simulink model "heli_model"  (R2025a)
settings: Solver=ode3  StartTime=0.0  StopTime=300  FixedStep=0.001
values from neighbouring files (symbols this model uses):
  alt = -1000    [Trim_Lin_Lqr.m]
  Vrefs = [15 20 25]    [Trim_Lin_Lqr.m]
  wp = [0 0; 1000 1000; 2000 0; 1000 -1000; 0 -100]    [Trim_Lin_Lqr.m]
undefined symbols (not defined in the file or in its folder): AngVel, AngVeltr, Coeffs, Lfin, LQR, MTOW, R, rad, Rtr, s
libraries: slpidlib x2, simulink x2, aerolibatmos2 x2, matrix_library x2, aerolibconvert2 x2, aerolibfltsims x2, aerolibsim3d x2, aerolibobsolete x1, sim3dlib x1
settings Model: PacingRate=1000  Creator=stand-alone1  LastModifiedBy=celal

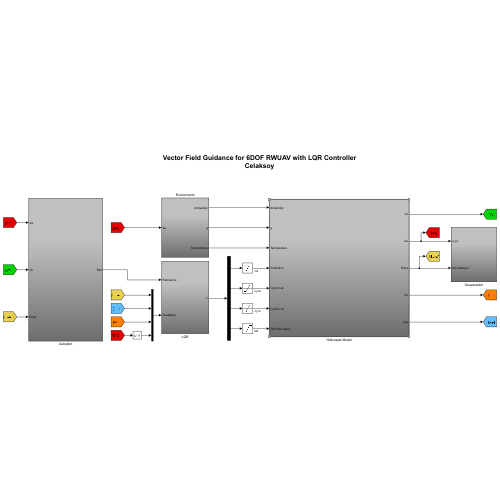
[thumbnail: Simulink's stored preview of the top-level diagram]
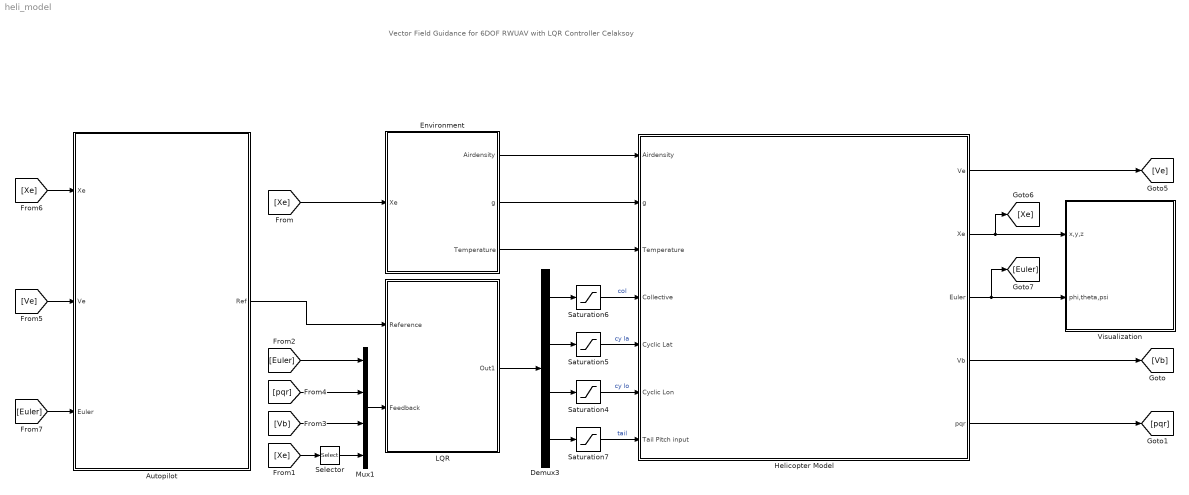
== system heli_model ==
  note: Vector Field Guidance for 6DOF RWUAV with LQR Controller
      | Celaksoy
  Autopilot : Subsystem
  Demux3 : Demux
  Environment : Subsystem
  Helicopter Model : Subsystem
  LQR : Subsystem
  Mux1 : Mux
  Saturation4 : Saturate  UpperLimit=0.25  LowerLimit=-0.25
  Saturation5 : Saturate  UpperLimit=0.25  LowerLimit=-0.25
  Saturation6 : Saturate  UpperLimit=0.15  LowerLimit=0.08
  Saturation7 : Saturate  LowerLimit=0
  Selector : Selector  InputPortWidth=3  IndexOptions=Index vector (dialog)  Indices=[3]  OutputSizes=1
  Visualization : Subsystem
  wires:
  Saturation4/1 -> Helicopter Model/6(Cyclic Lon)  "cy lo"
  Saturation5/1 -> Helicopter Model/5(Cyclic Lat)  "cy la"
  Saturation7/1 -> Helicopter Model/7(Tail Pitch input)  "tail"
  Demux3/1 -> Saturation6/1
  Demux3/2 -> Saturation5/1
  Demux3/4 -> Saturation7/1
  Demux3/3 -> Saturation4/1
  Saturation6/1 -> Helicopter Model/4(Collective)  "col"
  LQR/1(Out1) -> Demux3/1
  Helicopter Model/2(Xe) -> Visualization/1(x,y,z), [Xe]
  Helicopter Model/3(Euler) -> Visualization/2(phi,theta,psi), [Euler]
  Helicopter Model/4(Vb) -> [Vb]
  Helicopter Model/5(pqr) -> [pqr]
  Helicopter Model/1(Ve) -> [Ve]
  Environment/1(Airdensity) -> Helicopter Model/1(Airdensity)
  Environment/2(g) -> Helicopter Model/2(g)
  Environment/3(Temperature) -> Helicopter Model/3(Temperature)
  [Xe] -> Environment/1(Xe)
  [Euler] -> Mux1/1
  [pqr] -> Mux1/2
  [Vb] -> Mux1/3
  [Xe] -> Selector/1
  Selector/1 -> Mux1/4
  Mux1/1 -> LQR/2(Feedback)
  Autopilot/1(Ref) -> LQR/1(Reference)
  [Xe] -> Autopilot/1(Xe)
  [Ve] -> Autopilot/2(Ve)
  [Euler] -> Autopilot/3(Euler)

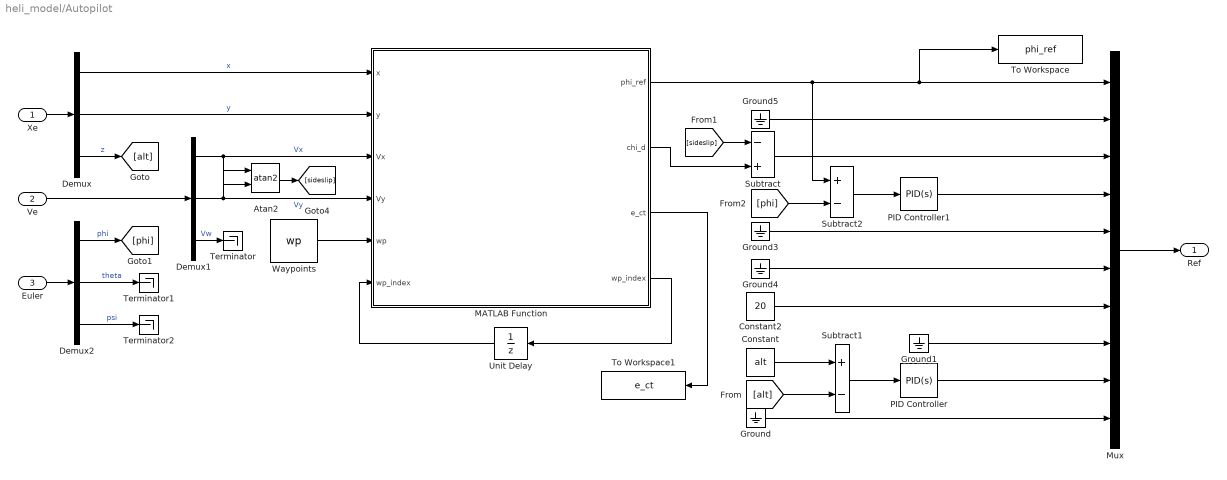
== system heli_model/Autopilot ==
  Xe : Inport
  Ve : Inport  Port=2
  Euler : Inport  Port=3
  Atan2 : Trigonometry  Operator=atan2
  Constant : Constant  Value=alt
  Constant2 : Constant  Value=20
  Demux : Demux  Outputs=3
  Demux1 : Demux  Outputs=3
  Demux2 : Demux  Outputs=3
  Ground{,1,3..5} (5 alike) : Ground
  MATLAB Function : MATLAB Function  TreatAsAtomicUnit=on
  Mux : Mux  Inputs=10
  PID Controller : slpidlib/PID Controller  Controller=PID  Form=Parallel  TimeDomain=Continuous-time  UseExternalTs=off  SampleTime=-1  IntegratorMethod=Forward Euler  FilterMethod=Forward Euler  ControllerParametersSource=internal  P=1  I=0.1  UseKiTs=off  D=0  UseExternalDerivativeSource=off  N=100  UseFilter=on  TunerSelectOption=Transfer Function Based (PID Tuner App)  InitialConditionSource=internal  InitialConditionForIntegrator=0  InitialConditionForFilter=0  DifferentiatorICPrevScaledInput=0  ExternalReset=none  TrackingMode=off  Kt=1  LimitOutput=off  SatLimitsSource=internal  UpperSaturationLimit=inf  LowerSaturationLimit=-inf  LinearizeAsGain=on  AntiWindupMode=none  Kb=1  LimitIntegrator=off  UpperIntegratorSaturationLimit=inf  LowerIntegratorSaturationLimit=-inf  POutMin=[]  POutMax=[]  IOutMin=[]  IOutMax=[]  DOutMin=[]  DOutMax=[]  NOutMin=[]  NOutMax=[]  SumOutMin=[]  SumOutMax=[]  SaturationOutMin=[]  SaturationOutMax=[]  PParamMin=[]  PParamMax=[]  IParamMin=[]  IParamMax=[]  DParamMin=[]  DParamMax=[]  NParamMin=[]  NParamMax=[]  KbParamMin=[]  KbParamMax=[]  KtParamMin=[]  KtParamMax=[]  KbOutMin=[]  KbOutMax=[]  KtOutMin=[]  KtOutMax=[]  IntegratorOutMin=[]  IntegratorOutMax=[]  FilterOutMin=[]  FilterOutMax=[]  SumI1OutMin=[]  SumI1OutMax=[]  SumI2OutMin=[]  SumI2OutMax=[]  SumI3OutMin=[]  SumI3OutMax=[]  SumI4OutMin=[]  SumI4OutMax=[]  SumDOutMin=[]  SumDOutMax=[]  DifferentiatorOutMin=[]  DifferentiatorOutMax=[]  FilterDiffOutCoefMin=[]  FilterDiffOutCoefMax=[]  ReciprocalOutMin=[]  ReciprocalOutMax=[]  SumDenOutMin=[]  SumDenOutMax=[]  SumNumOutMin=[]  SumNumOutMax=[]  DivideOutMin=[]  DivideOutMax=[]  UdiffTsProdOutMin=[]  UdiffTsProdOutMax=[]  NTsProdOutMin=[]  NTsProdOutMax=[]  UintegralTsProdOutMin=[]  UintegralTsProdOutMax=[]  UngainTsProdOutMin=[]  UngainTsProdOutMax=[]  ClampingZeroOutDataTypeStr=Inherit: Inherit via back propagation  ClampingZeroOutMin=[]  ClampingZeroOutMax=[]  FilterDenConstantOutDataTypeStr=Inherit: Inherit via back propagation  FilterDenConstantOutMin=[]  FilterDenConstantOutMax=[]  PCopyOutDataTypeStr=Inherit: Inherit via back propagation  PCopyOutMin=[]  PCopyOutMax=[]  NCopyOutDataTypeStr=Inherit: Inherit via back propagation  NCopyOutMin=[]  NCopyOutMax=[]  IntegratorContinuousStateAttributes=''  IntegratorStateMustResolveToSignalObject=off  IntegratorRTWStateStorageClass=Auto  FilterContinuousStateAttributes=''  FilterStateMustResolveToSignalObject=off  FilterRTWStateStorageClass=Auto  ParallelPVariant=InternalParameters  IdealPVariant=Disabled  IVariant=InternalParameters  DVariant=InternalParameters  IntegratorVariant=Continuous  SatVariant=Disabled  AWVariant=Passthrough  PCopyVariant=Disabled  TRVariant=Disabled  FdbkBlocksVariant=Forward  IdealPFdbkVariant=Disabled  SatFdbkVariant=Disabled  DerivativeFilterVariant=ContFilter  NVariant=InternalParameters  NCopyVariant=Disabled  FilterICVariant=InternalICsFilter  IntegratorICVariant=InternalICs  ExternalResetVariant=Disabled  TRSumVariant=Passthrough  SumFdbkVariant=Disabled  SumVariant=Sum_PID  TsampFilterVariant=InternalTs  TsampNgainVariant=Passthrough  TsampIntegralVariant=Disabled_SignalSpec  ExternalSaturationOutDataTypeStr=Inherit: Same as second input  DerivativeSourceVariant=ErrorSignal  PreIntVariant=InternalPreInt
  PID Controller1 : slpidlib/PID Controller  Controller=PID  Form=Parallel  TimeDomain=Continuous-time  UseExternalTs=off  SampleTime=-1  IntegratorMethod=Forward Euler  FilterMethod=Forward Euler  ControllerParametersSource=internal  P=1  I=0.1  UseKiTs=off  D=0  UseExternalDerivativeSource=off  N=100  UseFilter=on  TunerSelectOption=Transfer Function Based (PID Tuner App)  InitialConditionSource=internal  InitialConditionForIntegrator=0  InitialConditionForFilter=0  DifferentiatorICPrevScaledInput=0  ExternalReset=none  TrackingMode=off  Kt=1  LimitOutput=off  SatLimitsSource=internal  UpperSaturationLimit=inf  LowerSaturationLimit=-inf  LinearizeAsGain=on  AntiWindupMode=none  Kb=1  LimitIntegrator=off  UpperIntegratorSaturationLimit=inf  LowerIntegratorSaturationLimit=-inf  POutMin=[]  POutMax=[]  IOutMin=[]  IOutMax=[]  DOutMin=[]  DOutMax=[]  NOutMin=[]  NOutMax=[]  SumOutMin=[]  SumOutMax=[]  SaturationOutMin=[]  SaturationOutMax=[]  PParamMin=[]  PParamMax=[]  IParamMin=[]  IParamMax=[]  DParamMin=[]  DParamMax=[]  NParamMin=[]  NParamMax=[]  KbParamMin=[]  KbParamMax=[]  KtParamMin=[]  KtParamMax=[]  KbOutMin=[]  KbOutMax=[]  KtOutMin=[]  KtOutMax=[]  IntegratorOutMin=[]  IntegratorOutMax=[]  FilterOutMin=[]  FilterOutMax=[]  SumI1OutMin=[]  SumI1OutMax=[]  SumI2OutMin=[]  SumI2OutMax=[]  SumI3OutMin=[]  SumI3OutMax=[]  SumI4OutMin=[]  SumI4OutMax=[]  SumDOutMin=[]  SumDOutMax=[]  DifferentiatorOutMin=[]  DifferentiatorOutMax=[]  FilterDiffOutCoefMin=[]  FilterDiffOutCoefMax=[]  ReciprocalOutMin=[]  ReciprocalOutMax=[]  SumDenOutMin=[]  SumDenOutMax=[]  SumNumOutMin=[]  SumNumOutMax=[]  DivideOutMin=[]  DivideOutMax=[]  UdiffTsProdOutMin=[]  UdiffTsProdOutMax=[]  NTsProdOutMin=[]  NTsProdOutMax=[]  UintegralTsProdOutMin=[]  UintegralTsProdOutMax=[]  UngainTsProdOutMin=[]  UngainTsProdOutMax=[]  ClampingZeroOutDataTypeStr=Inherit: Inherit via back propagation  ClampingZeroOutMin=[]  ClampingZeroOutMax=[]  FilterDenConstantOutDataTypeStr=Inherit: Inherit via back propagation  FilterDenConstantOutMin=[]  FilterDenConstantOutMax=[]  PCopyOutDataTypeStr=Inherit: Inherit via back propagation  PCopyOutMin=[]  PCopyOutMax=[]  NCopyOutDataTypeStr=Inherit: Inherit via back propagation  NCopyOutMin=[]  NCopyOutMax=[]  IntegratorContinuousStateAttributes=''  IntegratorStateMustResolveToSignalObject=off  IntegratorRTWStateStorageClass=Auto  FilterContinuousStateAttributes=''  FilterStateMustResolveToSignalObject=off  FilterRTWStateStorageClass=Auto  ParallelPVariant=InternalParameters  IdealPVariant=Disabled  IVariant=InternalParameters  DVariant=InternalParameters  IntegratorVariant=Continuous  SatVariant=Disabled  AWVariant=Passthrough  PCopyVariant=Disabled  TRVariant=Disabled  FdbkBlocksVariant=Forward  IdealPFdbkVariant=Disabled  SatFdbkVariant=Disabled  DerivativeFilterVariant=ContFilter  NVariant=InternalParameters  NCopyVariant=Disabled  FilterICVariant=InternalICsFilter  IntegratorICVariant=InternalICs  ExternalResetVariant=Disabled  TRSumVariant=Passthrough  SumFdbkVariant=Disabled  SumVariant=Sum_PID  TsampFilterVariant=InternalTs  TsampNgainVariant=Passthrough  TsampIntegralVariant=Disabled_SignalSpec  ExternalSaturationOutDataTypeStr=Inherit: Same as second input  DerivativeSourceVariant=ErrorSignal  PreIntVariant=InternalPreInt
  Subtract : Sum  Inputs=-+
  Subtract1 : Sum  Inputs=+-
  Subtract2 : Sum  Inputs=+-
  Terminator : Terminator
  Terminator1 : Terminator
  Terminator2 : Terminator
  To Workspace : ToWorkspace  VariableName=phi_ref  SaveFormat=Timeseries  SampleTime=-1
  To Workspace1 : ToWorkspace  VariableName=e_ct  SaveFormat=Timeseries  SampleTime=-1
  Unit Delay : UnitDelay  InitialCondition=1  SampleTime=-1  HasFrameUpgradeWarning=on
  Waypoints : Constant  Value=wp
  Ref : Outport
  wires:
  MATLAB Function/4(wp_index) -> Unit Delay/1
  Waypoints/1 -> MATLAB Function/5(wp)
  Unit Delay/1 -> MATLAB Function/6("wp_index ")
  Xe/1 -> Demux/1
  Demux/1 -> MATLAB Function/1(x)  "x"
  Demux/2 -> MATLAB Function/2(y)  "y"
  Demux/3 -> [alt]  "z"
  Ve/1 -> Demux1/1
  Demux1/1 -> MATLAB Function/3(Vx), Atan2/2  "Vx"
  Demux1/2 -> MATLAB Function/4(Vy), Atan2/1  "Vy"
  Euler/1 -> Demux2/1
  Demux1/3 -> Terminator/1  "Vw"
  Demux2/1 -> [phi]  "phi"
  Demux2/2 -> Terminator1/1  "theta"
  Demux2/3 -> Terminator2/1  "psi"
  MATLAB Function/1(phi_ref) -> To Workspace/1, Mux/1, Subtract2/1
  Atan2/1 -> [sideslip]
  MATLAB Function/2(chi_d) -> Subtract/2
  [sideslip] -> Subtract/1
  Mux/1 -> Ref/1
  Constant2/1 -> Mux/7
  Subtract/1 -> Mux/3
  Ground5/1 -> Mux/2
  Ground/1 -> Mux/10
  Constant/1 -> Subtract1/1
  [alt] -> Subtract1/2
  Subtract1/1 -> PID Controller/1
  PID Controller/1 -> Mux/9
  Ground1/1 -> Mux/8
  Ground4/1 -> Mux/6
  Ground3/1 -> Mux/5
  [phi] -> Subtract2/2
  Subtract2/1 -> PID Controller1/1
  PID Controller1/1 -> Mux/4
  MATLAB Function/3(e_ct) -> To Workspace1/1

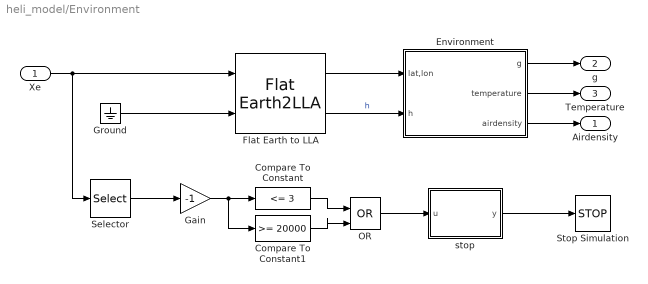
== system heli_model/Environment ==
  Xe : Inport
  Compare To Constant : simulink/Logic and Bit Operations/Compare To Constant  relop=<=  const=3  OutDataTypeStr=boolean
  Compare To Constant1 : simulink/Logic and Bit Operations/Compare To Constant  relop=>=  const=20000  OutDataTypeStr=boolean
  Environment : Subsystem  mask{atmomodel=ISA, consg=on}
      mask prompts: atmomodel "Atmosphere Model"; consg "Constant g (Gravitational Acceleration)"
      mask DialogControl a Prompt: Environment
      mask DialogControl b Prompt: Wind simulation, atmosphere properties and gravity model
      mask DialogControl Container4 Prompt: Environment
  Flat Earth to LLA : FlatEarth2LLA  R=6378137
  Gain : Gain  Gain=-1
  Ground : Ground
  OR : Logic  Operator=OR  IconShape=distinctive  AllPortsSameDT=off  OutDataTypeStr=boolean
  Selector : Selector  InputPortWidth=3  IndexOptions=Index vector (dialog)  Indices=[3]  OutputSizes=1
  Stop Simulation : Stop
  stop : MATLAB Function  TreatAsAtomicUnit=on
  Airdensity : Outport
  g : Outport  Port=2
  Temperature : Outport  Port=3
  wires:
  Compare To Constant/1 -> OR/1
  OR/1 -> stop/1(u)
  stop/1(y) -> Stop Simulation/1
  Compare To Constant1/1 -> OR/2
  Gain/1 -> Compare To Constant1/1, Compare To Constant/1
  Ground/1 -> Flat Earth to LLA/2
  Flat Earth to LLA/1 -> Environment/1(lat,lon)
  Flat Earth to LLA/2 -> Environment/2(h)  "h"
  Xe/1 -> Selector/1, Flat Earth to LLA/1
  Selector/1 -> Gain/1
  Environment/1(g) -> g/1
  Environment/2(temperature) -> Temperature/1
  Environment/3(airdensity) -> Airdensity/1

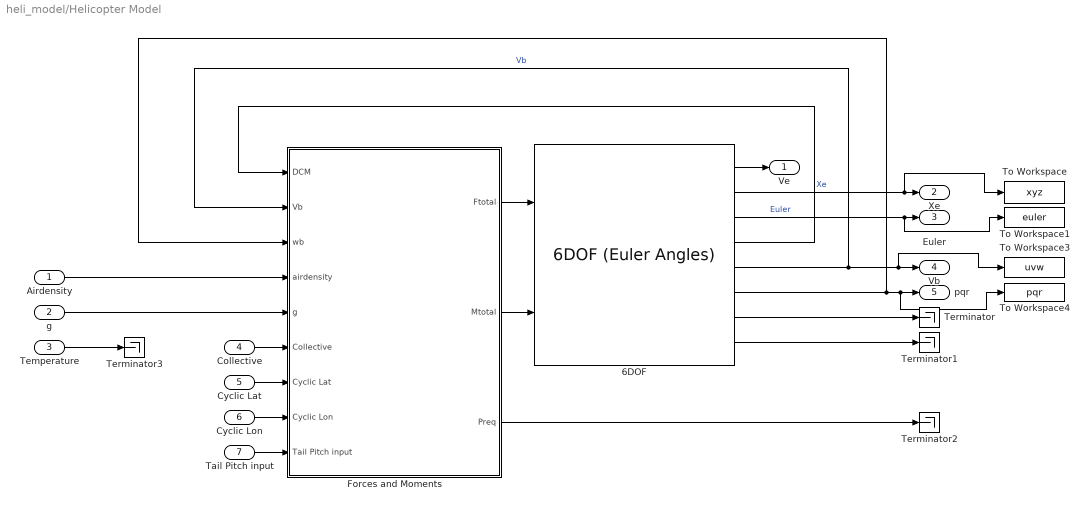
== system heli_model/Helicopter Model ==
  Airdensity : Inport
  g : Inport  Port=2
  Temperature : Inport  Port=3
  Collective : Inport  Port=4
  Cyclic Lat : Inport  Port=5
  Cyclic Lon : Inport  Port=6
  Tail Pitch input : Inport  Port=7
  6DOF : aerolibobsolete/6DOF (Euler Angles)  units=Metric (MKS)  mtype=Fixed  rep=Euler Angles  xme_0=[0;0;-1000]  Vm_0=[20;0;0]  eul_0=[0;0;0]  pm_0=[0;0;0]  mass_0=MTOW  mass_e=0.5  mass_f=2.0  inertia=|  inertia_e=eye(3)  inertia_f=2*eye(3)  k_quat=1.0  vre_flag=off  abi_flag=off  aMode=0  xme_statename=''  Vm_statename=''  eul_statename=''  quat_statename=''  pm_statename=''  mass_statename=''
      | [Inertias(1) 0 0; 0 Inertias(2) 0;
      | 0 0 Inertias(3)];
  Forces and Moments : Subsystem
  Terminator{,1..3} (4 alike) : Terminator
  To Workspace : ToWorkspace  VariableName=xyz  SaveFormat=Timeseries  SampleTime=-1
  To Workspace1 : ToWorkspace  VariableName=euler  SaveFormat=Timeseries  SampleTime=-1
  To Workspace3 : ToWorkspace  VariableName=uvw  SaveFormat=Timeseries  SampleTime=-1
  To Workspace4 : ToWorkspace  VariableName=pqr  SaveFormat=Timeseries  SampleTime=-1
  Ve : Outport
  Xe : Outport  Port=2
  Euler : Outport  Port=3
  Vb : Outport  Port=4
  pqr : Outport  Port=5
  wires:
  6DOF/1 -> Ve/1
  6DOF/8 -> Terminator1/1
  Forces and Moments/1(Ftotal) -> 6DOF/1
  Forces and Moments/2(Mtotal) -> 6DOF/2
  6DOF/6 -> Forces and Moments/3(wb), To Workspace4/1, pqr/1
  6DOF/4 -> Forces and Moments/1(DCM)
  6DOF/7 -> Terminator/1
  6DOF/5 -> Forces and Moments/2(Vb), To Workspace3/1, Vb/1  "Vb"
  Cyclic Lat/1 -> Forces and Moments/7(Cyclic Lat)
  Collective/1 -> Forces and Moments/6(Collective)
  6DOF/3 -> To Workspace1/1, Euler/1  "Euler"
  Tail Pitch input/1 -> Forces and Moments/9(Tail Pitch input)
  Cyclic Lon/1 -> Forces and Moments/8(Cyclic Lon)
  g/1 -> Forces and Moments/5(g)
  6DOF/2 -> To Workspace/1, Xe/1  "Xe"
  Airdensity/1 -> Forces and Moments/4(airdensity)
  Forces and Moments/3(Preq) -> Terminator2/1
  Temperature/1 -> Terminator3/1

== system heli_model/LQR ==
  Reference : Inport
  Feedback : Inport  Port=2
  Constant4 : Constant  Value=LQR.K_lqr
  Constant5 : Constant  Value=Vrefs
  Gain : Gain  Gain=-1
  MATLAB Function : MATLAB Function  TreatAsAtomicUnit=on
  MatrixMultiply : Product  Multiplication=Matrix(*)
  Selector1 : Selector  InputPortWidth=10  IndexOptions=Index vector (dialog)  Indices=[7]  OutputSizes=1
  Sum1 : Sum  Inputs=|+-
  Out1 : Outport
  wires:
  Gain/1 -> MatrixMultiply/1
  Sum1/1 -> MatrixMultiply/2
  Selector1/1 -> MATLAB Function/1(u)
  Constant4/1 -> MATLAB Function/2(K_table)
  Constant5/1 -> MATLAB Function/3(Vrefs)
  MatrixMultiply/1 -> Out1/1
  Reference/1 -> Sum1/2
  Feedback/1 -> Sum1/1, Selector1/1
  MATLAB Function/1(K) -> Gain/1

== system heli_model/Visualization ==
  x,y,z : Inport
  phi,theta,psi : Inport  Port=2
  Demux : Demux  Outputs=2
  Demux1 : Demux  Outputs=3
  Flat Earth to LLA : FlatEarth2LLA  R=6378137
  FlightGear Preconfigured 6DoF Animation : aerolibfltsims/FlightGear Preconfigured 6DoF Animation  xFlightGearVersion=v2019.1  DestinationIpAddress=127.0.0.1  DestinationPort=5502  SampleTime=-1  packetVersion=24
  "Generate Run Script " : aerolibfltsims/Generate Run Script  Architecture=Default  dataFlow=Send  GeometryModelName=c172p  AirportId=KSFO  RunwayId=10L  InitialAltitude=7224  InitialHeading=113  OffsetDistance=4.72  OffsetAzimuth=0  InstallScenery=off  DisableShaders=on  OriginAddress=127.0.0.1  DestinationPort=5502  OriginPort=5505  LocalAddress=127.0.0.1  OutputFileName=runFlightGear.bat  FlightGearBaseDirectory=C:\Program Files\FlightGear 2020.3
  Ground : Ground
  Mux : Mux  Inputs=6
  Mux1 : Mux  Inputs=2
  Variant Subsystem : Subsystem  Variant=on
  wires:
  phi,theta,psi/1 -> Demux1/1, Mux1/2
  Demux1/3 -> Mux/6  "psi"
  Demux1/2 -> Mux/5  "theta"
  Demux1/1 -> Mux/4  "phi"
  Flat Earth to LLA/2 -> Mux/3  "h"
  Mux/1 -> FlightGear Preconfigured 6DoF Animation/1
  Demux/1 -> Mux/2  "mu"
  Demux/2 -> Mux/1  "l"
  Flat Earth to LLA/1 -> Demux/1
  Mux1/1 -> Variant Subsystem/1(states)
  Ground/1 -> Flat Earth to LLA/2
  x,y,z/1 -> Flat Earth to LLA/1, Mux1/1

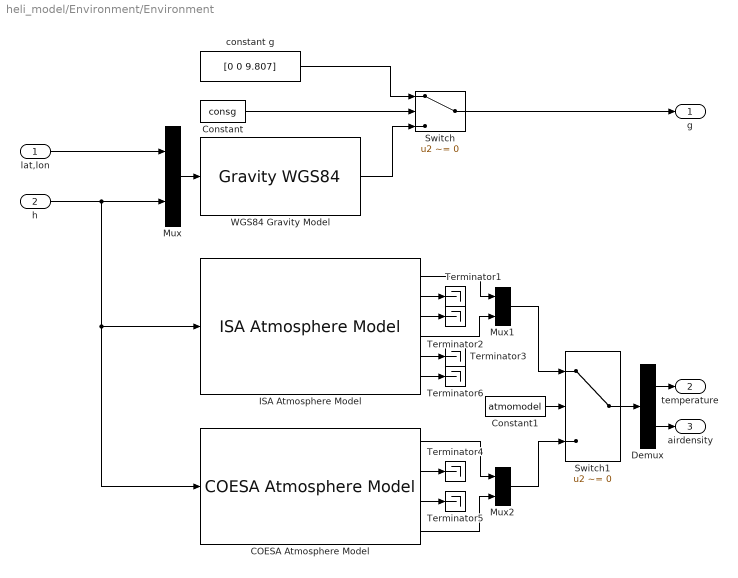
== system heli_model/Environment/Environment ==
  lat,lon : Inport
  h : Inport  Port=2
  COESA Atmosphere Model : aerolibatmos2/COESA Atmosphere Model  units=Metric (MKS)  spec=1976 COESA-extended U.S. Standard Atmosphere  model=Profile  profile_var=High temperature  profile_percent=1%  profile_alt=5 km (16404 ft)  envelope_var=High temperature  envelope_percent=1%  action=Warning
  Constant : Constant  Value=consg
  Constant1 : Constant  Value=atmomodel
  Demux : Demux  Outputs=2
  ISA Atmosphere Model : aerolibatmos2/ISA Atmosphere Model  useExtended=off  action=Warning  custom=off  viscosityOut=on  g=9.80665  gamma=1.4  R=287.0531  L=0.0065  h_trop=11000  h_strat=20000  rho0=1.225  P0=101325  T0=288.15  h0=0  S=110.4  Tref=273.15  muref=1.716e-5
  Mux : Mux  Inputs=2
  Mux1 : Mux  Inputs=2
  Mux2 : Mux  Inputs=2
  Switch : Switch  Criteria=u2 ~= 0  SaturateOnIntegerOverflow=off  InputSameDT=off
  Switch1 : Switch  Criteria=u2 ~= 0  SaturateOnIntegerOverflow=off  InputSameDT=off
  Terminator{1..6} (6 alike) : Terminator
  "WGS84 Gravity Model  " : GravityWGS84
  constant g : Constant  Value=[0 0 9.807]
  g : Outport
  temperature : Outport  Port=2
  airdensity : Outport  Port=3
  wires:
  lat,lon/1 -> Mux/1
  Constant/1 -> Switch/2
  constant g/1 -> Switch/1
  "WGS84 Gravity Model  "/1 -> Switch/3
  Switch/1 -> g/1
  Mux/1 -> "WGS84 Gravity Model  "/1
  h/1 -> COESA Atmosphere Model/1, ISA Atmosphere Model/1, Mux/2
  Switch1/1 -> Demux/1
  ISA Atmosphere Model/1 -> Mux1/1
  ISA Atmosphere Model/2 -> Terminator1/1
  ISA Atmosphere Model/3 -> Terminator2/1
  COESA Atmosphere Model/2 -> Terminator4/1
  COESA Atmosphere Model/1 -> Mux2/1
  COESA Atmosphere Model/3 -> Terminator5/1
  ISA Atmosphere Model/4 -> Mux1/2
  COESA Atmosphere Model/4 -> Mux2/2
  Constant1/1 -> Switch1/2
  Mux1/1 -> Switch1/1
  Mux2/1 -> Switch1/3
  Demux/2 -> airdensity/1
  Demux/1 -> temperature/1
  ISA Atmosphere Model/5 -> Terminator3/1
  ISA Atmosphere Model/6 -> Terminator6/1

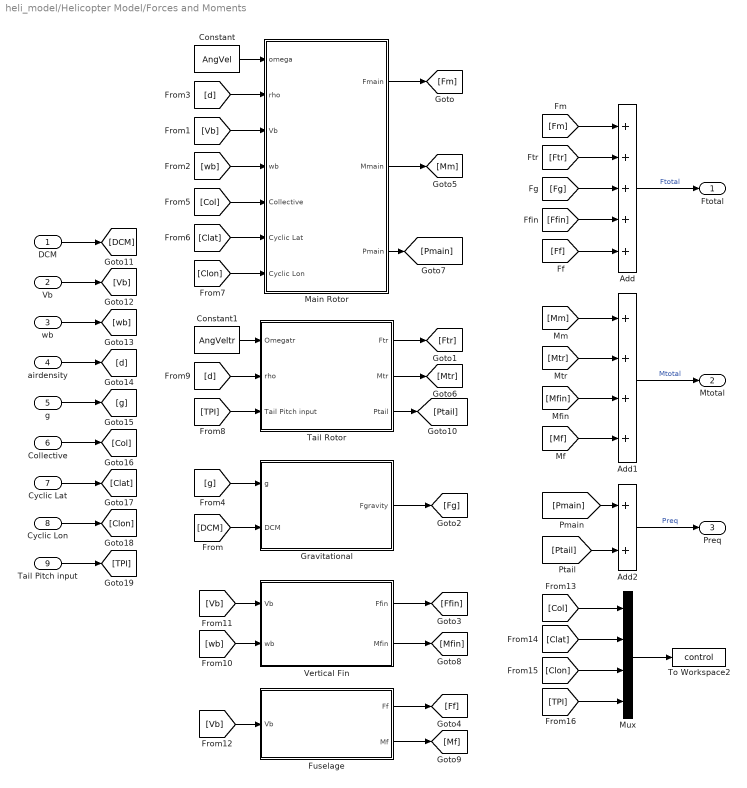
== system heli_model/Helicopter Model/Forces and Moments ==
  DCM : Inport
  Vb : Inport  Port=2
  wb : Inport  Port=3
  airdensity : Inport  Port=4
  g : Inport  Port=5
  Collective : Inport  Port=6
  Cyclic Lat : Inport  Port=7
  Cyclic Lon : Inport  Port=8
  Tail Pitch input : Inport  Port=9
  Add : Sum  Inputs=+++++
  Add1 : Sum  Inputs=++++
  Add2 : Sum
  Constant : Constant  Value=AngVel
  Constant1 : Constant  Value=AngVeltr
  Fuselage : Subsystem
  Gravitational : Subsystem
  Main Rotor : Subsystem
  Mux : Mux
  Tail Rotor : Subsystem
  To Workspace2 : ToWorkspace  VariableName=control  SaveFormat=Timeseries  SampleTime=-1
  Vertical Fin : Subsystem
  Ftotal : Outport
  Mtotal : Outport  Port=2
  Preq : Outport  Port=3
  wires:
  Add/1 -> Ftotal/1  "Ftotal"
  Main Rotor/1(Fmain) -> [Fm]
  Tail Rotor/1(Ftr) -> [Ftr]
  Gravitational/1(Fgravity) -> [Fg]
  Vertical Fin/1(Ffin) -> [Ffin]
  [Fm] -> Add/1
  [Ftr] -> Add/2
  [Fg] -> Add/3
  [Ffin] -> Add/4
  [Ff] -> Add/5
  Main Rotor/2(Mmain) -> [Mm]
  Tail Rotor/2(Mtr) -> [Mtr]
  Vertical Fin/2(Mfin) -> [Mfin]
  [Mm] -> Add1/1
  [Mtr] -> Add1/2
  [Mf] -> Add1/4
  [Mfin] -> Add1/3
  Constant/1 -> Main Rotor/1(omega)
  Constant1/1 -> Tail Rotor/1(Omegatr)
  Add2/1 -> Preq/1  "Preq"
  Main Rotor/3(Pmain) -> [Pmain]
  Tail Rotor/3(Ptail) -> [Ptail]
  [Pmain] -> Add2/1
  [Ptail] -> Add2/2
  Fuselage/1(Ff) -> [Ff]
  Fuselage/2(Mf) -> [Mf]
  Add1/1 -> Mtotal/1  "Mtotal"
  DCM/1 -> [DCM]
  Vb/1 -> [Vb]
  wb/1 -> [wb]
  airdensity/1 -> [d]
  g/1 -> [g]
  Collective/1 -> [Col]
  Cyclic Lat/1 -> [Clat]
  Cyclic Lon/1 -> [Clon]
  Tail Pitch input/1 -> [TPI]
  [d] -> Main Rotor/2(rho)
  [Vb] -> Main Rotor/3(Vb)
  [wb] -> Main Rotor/4(wb)
  [Col] -> Main Rotor/5(Collective)
  [Clat] -> Main Rotor/6(Cyclic Lat)
  [Clon] -> Main Rotor/7(Cyclic Lon)
  [d] -> Tail Rotor/2(rho)
  [TPI] -> Tail Rotor/3(Tail Pitch input)
  [g] -> Gravitational/1(g)
  [DCM] -> Gravitational/2(DCM)
  [Vb] -> Vertical Fin/1(Vb)
  [Vb] -> Fuselage/1(Vb)
  [wb] -> Vertical Fin/2(wb)
  [Col] -> Mux/1
  [Clat] -> Mux/2
  [Clon] -> Mux/3
  [TPI] -> Mux/4
  Mux/1 -> To Workspace2/1

== system heli_model/Visualization/Variant Subsystem ==
  note: Set visual = true to visualize using Simulink 3D Animation and
      | visual = false to visualize scope results without enabling Simulink 3D Animation
  states : Inport
  Simulink 3D Animation : Subsystem  VariantControl=(default)

== system heli_model/Helicopter Model/Forces and Moments/Fuselage ==
  Vb : Inport
  Demux : Demux  Outputs=3
  Fuselage Forces : Subsystem
  Fuselage Moments : Subsystem
  Ff : Outport
  Mf : Outport  Port=2
  wires:
  Demux/1 -> Fuselage Forces/1(u), Fuselage Moments/1(u)
  Demux/2 -> Fuselage Moments/2(v), Fuselage Forces/2(v)
  Demux/3 -> Fuselage Moments/3(w), Fuselage Forces/3(w)
  Vb/1 -> Demux/1
  Fuselage Moments/1(Mf) -> Mf/1
  Fuselage Forces/1(Ff) -> Ff/1

== system heli_model/Helicopter Model/Forces and Moments/Gravitational ==
  g : Inport
  DCM : Inport  Port=2
  Constant : Constant  Value=MTOW
  MatrixMultiply : Product  Multiplication=Matrix(*)
  Product : Product
  Fgravity : Outport
  wires:
  DCM/1 -> MatrixMultiply/1
  MatrixMultiply/1 -> Fgravity/1
  Product/1 -> MatrixMultiply/2
  Constant/1 -> Product/2
  g/1 -> Product/1

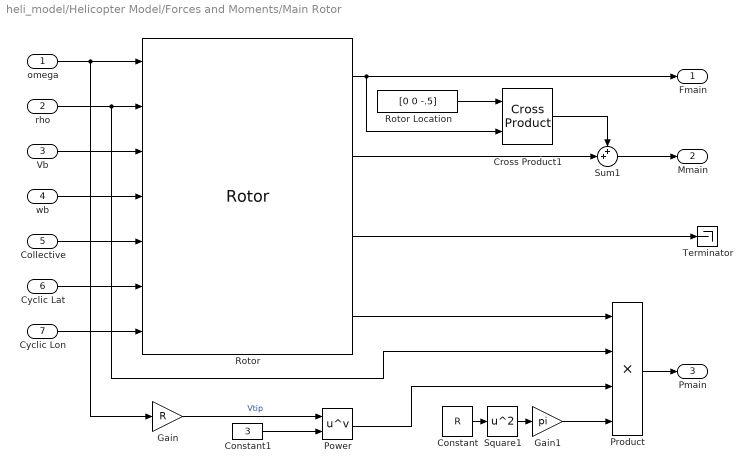
== system heli_model/Helicopter Model/Forces and Moments/Main Rotor ==
  omega : Inport
  rho : Inport  Port=2
  Vb : Inport  Port=3
  wb : Inport  Port=4
  Collective : Inport  Port=5
  Cyclic Lat : Inport  Port=6
  Cyclic Lon : Inport  Port=7
  Constant : Constant  Value=R
  Constant1 : Constant  Value=3
  Cross Product1 : matrix_library/Cross Product
  Gain : Gain  Gain=R
  Gain1 : Gain  Gain=pi
  Power : Math  Operator=pow
  Product : Product  Inputs=4
  Rotor : Rotor  modelMode=With flap effects  controlInput=on  CTCQMode=Compute using BEMT  Nb=Nb  CTout=on  radius=R  chord=c  clalpha=CL_a  cd0=0.009  gamma=lockNum  thetaRoot=rootang  thetaTwist=twistang
  Rotor Location : Constant  Value=[0 0 -.5]  VectorParams1D=off
  Square1 : Math  Operator=square
  Sum1 : Sum  Inputs=++|
  Terminator : Terminator
  Fmain : Outport
  Mmain : Outport  Port=2
  Pmain : Outport  Port=3
  wires:
  omega/1 -> Gain/1, Rotor/1
  rho/1 -> Rotor/2, Product/2
  Rotor/3 -> Terminator/1
  Rotor/4 -> Product/1
  Cyclic Lon/1 -> Rotor/7
  Cyclic Lat/1 -> Rotor/6
  Vb/1 -> Rotor/3
  wb/1 -> Rotor/4
  Power/1 -> Product/3
  Gain/1 -> Power/1  "Vtip"
  Constant/1 -> Square1/1
  Square1/1 -> Gain1/1
  Gain1/1 -> Product/4
  Constant1/1 -> Power/2
  Product/1 -> Pmain/1
  Sum1/1 -> Mmain/1
  Rotor/1 -> Cross Product1/2, Fmain/1
  Rotor/2 -> Sum1/2
  Collective/1 -> Rotor/5
  Cross Product1/1 -> Sum1/1
  Rotor Location/1 -> Cross Product1/1

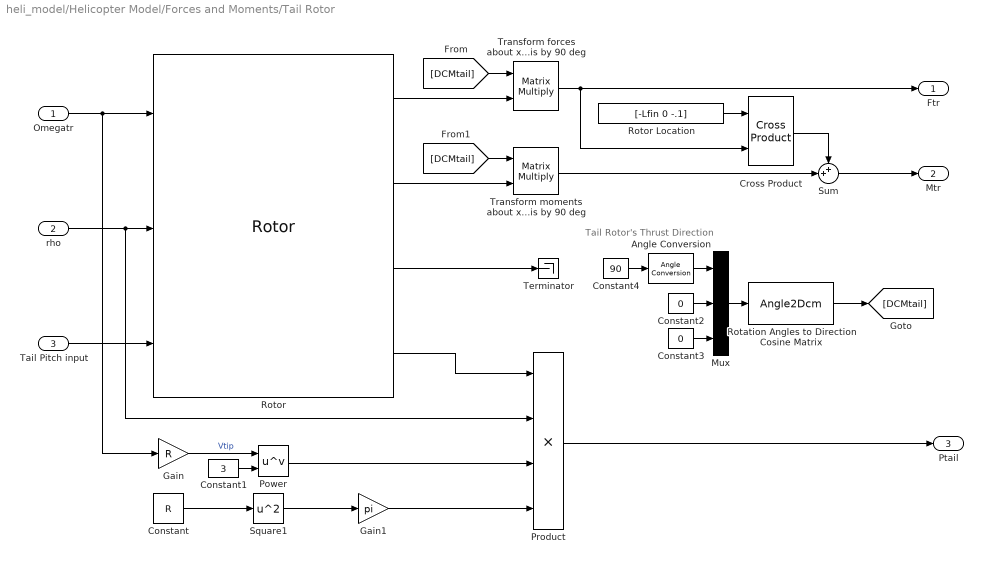
== system heli_model/Helicopter Model/Forces and Moments/Tail Rotor ==
  note: Tail Rotor's Thrust Direction
  Omegatr : Inport
  rho : Inport  Port=2
  Tail Pitch input : Inport  Port=3
  Angle Conversion : aerolibconvert2/Angle Conversion  IU=deg  OU=rad
  Constant : Constant  Value=R
  Constant1 : Constant  Value=3
  Constant2 : Constant  Value=0
  Constant3 : Constant  Value=0
  Constant4 : Constant  Value=90
  Cross Product : matrix_library/Cross Product
  Gain : Gain  Gain=R
  Gain1 : Gain  Gain=pi
  Mux : Mux  Inputs=3
  Power : Math  Operator=pow
  Product : Product  Inputs=4
  Rotation Angles to Direction Cosine Matrix : Angle2Dcm  rotationOrder=XYZ
      settings: AttributesFormatString=Rotation Order: %<rotationOrder>
  Rotor : Rotor  controlInput=on  CTCQMode=Compute using BEMT  Nb=Nbtr  CTout=on  radius=Rtr+.1  chord=0.12  cd0=0.009  thetaRoot=0.0001  thetaTwist=0.0001
  Rotor Location : Constant  Value=[-Lfin 0 -.1]  VectorParams1D=off
  Square1 : Math  Operator=square
  Sum : Sum  Inputs=++|
  Terminator : Terminator
  "Transform forces about x-axis by 90 deg " : Product  Multiplication=Matrix(*)
  Transform moments about x-axis by 90 deg : Product  Multiplication=Matrix(*)
  Ftr : Outport
  Mtr : Outport  Port=2
  Ptail : Outport  Port=3
  wires:
  Rotor/3 -> Terminator/1
  Tail Pitch input/1 -> Rotor/3
  Power/1 -> Product/3
  Constant1/1 -> Power/2
  Gain/1 -> Power/1  "Vtip"
  rho/1 -> Product/2, Rotor/2
  Rotor/4 -> Product/1
  Gain1/1 -> Product/4
  Omegatr/1 -> Gain/1, Rotor/1
  Square1/1 -> Gain1/1
  Constant/1 -> Square1/1
  Product/1 -> Ptail/1
  Rotor/2 -> Transform moments about x-axis by 90 deg/2
  Sum/1 -> Mtr/1
  Rotor Location/1 -> Cross Product/1
  Constant4/1 -> Angle Conversion/1
  Transform moments about x-axis by 90 deg/1 -> Sum/2
  Mux/1 -> Rotation Angles to Direction Cosine Matrix/1
  Angle Conversion/1 -> Mux/1
  Constant2/1 -> Mux/2
  Rotor/1 -> "Transform forces about x-axis by 90 deg "/2
  "Transform forces about x-axis by 90 deg "/1 -> Cross Product/2, Ftr/1
  Cross Product/1 -> Sum/1
  Constant3/1 -> Mux/3
  Rotation Angles to Direction Cosine Matrix/1 -> [DCMtail]
  [DCMtail] -> "Transform forces about x-axis by 90 deg "/1
  [DCMtail] -> Transform moments about x-axis by 90 deg/1

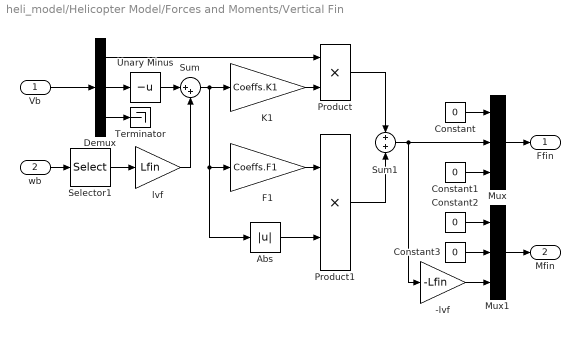
== system heli_model/Helicopter Model/Forces and Moments/Vertical Fin ==
  Vb : Inport
  wb : Inport  Port=2
  -lvf : Gain  Gain=-Lfin
  Abs : Abs  SaturateOnIntegerOverflow=off
  Constant{,1..3} (4 alike) : Constant  Value=0
  Demux : Demux  Outputs=3
  F1 : Gain  Gain=Coeffs.F1
  K1 : Gain  Gain=Coeffs.K1
  Mux : Mux  Inputs=3
  Mux1 : Mux  Inputs=3
  Product : Product
  Product1 : Product
  Selector1 : Selector  InputPortWidth=3  IndexOptions=Index vector (dialog)  Indices=[3]  OutputSizes=1
  Sum : Sum  Inputs=|++
  Sum1 : Sum  Inputs=+|+
  Terminator : Terminator
  Unary Minus : UnaryMinus
  lvf : Gain  Gain=Lfin
  Ffin : Outport
  Mfin : Outport  Port=2
  wires:
  Vb/1 -> Demux/1
  Unary Minus/1 -> Sum/1
  wb/1 -> Selector1/1
  Selector1/1 -> lvf/1
  lvf/1 -> Sum/2
  Demux/2 -> Unary Minus/1
  Demux/1 -> Product/1
  K1/1 -> Product/2
  F1/1 -> Product1/1
  Sum/1 -> F1/1, Abs/1, K1/1
  Abs/1 -> Product1/2
  Demux/3 -> Terminator/1
  Mux/1 -> Ffin/1
  Mux1/1 -> Mfin/1
  Constant/1 -> Mux/1
  Constant1/1 -> Mux/3
  Constant3/1 -> Mux1/2
  Constant2/1 -> Mux1/1
  Product/1 -> Sum1/1
  Product1/1 -> Sum1/2
  Sum1/1 -> -lvf/1, Mux/2
  -lvf/1 -> Mux1/3

== system heli_model/Visualization/Variant Subsystem/Simulink 3D Animation ==
  states : Inport
  Add : Sum
  Constant10 : Constant  Value=[5000 0 0]  VectorParams1D=off
  Demux : Demux  Outputs=2
  Simulation 3D Light Helicopter Pack : aerolibsim3d/Simulation 3D Light Helicopter Pack  Engine_T=off  Engine_R=off  Rotor1_T=off  Rotor1_R=on  Rotor2_T=off  Rotor2_R=on  Sensor1_T=off  Sensor1_R=off  Sensor2_T=off  Sensor2_R=off  GeoRadioButton=NED
      settings: AttributesFormatString=NED
  Simulation 3D Rotorcraft : aerolibsim3d/Simulation 3D Rotorcraft  Priority=-1  Mesh=Light helicopter  MeshPath=/MathWorksAerospaceContent/Vehicles/Rotorcraft/Helicopter/Mesh/SK_Helicopter.SK_Helicopter  MeshPathLight=/MathWorksAerospaceContent/Vehicles/Rotorcraft/LightHelicopter/Mesh/SK_LightHelicopter.SK_LightHelicopter  MeshPathMulti=/MathWorksAerospaceContent/Vehicles/Rotorcraft/Multirotor/Mesh/SK_Quadcopter.SK_Quadcopter  AircraftColor=Blue  ActorName=SimulinkVehicle1  Translation=[5000 0 -0.06;zeros(5,3)]  Rotation=zeros(6, 3)  ScaleInputPort=Dialog  Scale=[1 1 1]  InitialScale=[1 1 1]  IsGHSensorEnabled=off  AreGHRaysVisible=off  IsOutputReshapeEnabled=off  GHRayLength=1524  GHBodyOffset=1.169  GHFrontTireRadius=0.196  GHLeftTireRadius=0.203  GHRightTireRadius=0.203  GHContactLocation1=[1.47 -1.04 1.169]  GHContactLocation2=[-1.24 -1.04 1.169]  GHContactLocation3=[-1.24 1.04 1.169]  GHContactLocation4=[1.47 1.04 1.169]  WoWSensorTolerance=0.05  LightsConfig=Automatic lights  LandingLightIntensity=300000  LandingLightConeAngle=15  LandingLightColor=[1 1 1]  HelicopterLeftLandingLightLocation=[0 0 0]  HelicopterLeftLandingLightOrientation=[0 0 0]  NoseLightIntensity=150000  NoseLightConeAngle=36  HelicopterNoseLightLocation=[0 0 0]  HelicopterNoseLightOrientation=[0 0 0]  NavLightIntensity=500  PositionLightIntensity=500  StrobeLightIntensity=5000  StrobeLightColor=[1 1 1]  StrobePeriod=1.5  StrobePulseWidth=6  BeaconLightIntensity=4000  BeaconLightColor=[1 0 0]  BeaconPeriod=1.5  BeaconPulseWidth=10  SampleTime=-1  ActorType=SimulinkVehicle  ID=1  aMode=0  ActorTag=SimulinkVehicle1
  Simulation 3D Scene Configuration : sim3dlib/Simulation 3D Scene Configuration  Priority=0  ProjectFormat=Default Scenes  SceneDesc=Empty Grass  ProjectName=C:\Program Files\MATLAB\R2025a\toolbox\shared\sim3d_projects\automotive_project_windows\UE\WindowsNoEditor\VehicleSimulation.exe  ScenePath=/Game/Maps/HwStrght  EnableOpenDRIVE=off  vehTagList={'Custom';'Scene Origin';'SimulinkVehicle1'}  vehTag=SimulinkVehicle1  AttachedCameraRelativeTranslation=[0 0 0]  FreeCameraDefaultInitialTranslation=[-6, 0, 2]  AttachedCameraRelativeRotation=[0 0 0]  FreeCameraDefaultInitialRotation=[0, -15, 0]  ViewpointName=Custom  FreeCameraInitialTranslation=[-6, 0, 2]  ViewpointTranslation=[0 0 0]  FreeCameraInitialRotation=[0, -15, 0]  ViewpointRotation=[0 0 0]  OpVisEn=off  Ts=.02  EnableWindow=on  EnableRemoteAccess=off  EnableWeather=off  SunAzimuth=90  SunAltitude=40.0  EnableGeospatialSun=off  Latitude=0  Longitude=0  Date=2023-01-01  Time=10:30:00  GeoTimeZone=-5.0  SunDaylightSaving=off  wind=1  clouds=10  EnableVolumetricClouds=off  CloudCoverage=0  CloudAltitude=6  fog=0  rain=0  RaindropsEffect=off  SnowDensity=30.0  EnableGeospatial=off  TilesetSource=Earth terrain  UseTrueOrigin=off  OriginHeight=200  OriginLatitude=40.744652  OriginLongitude=-73.988864  MapStyle=Aerial  AdditionalAssetIDs=[]  UseAdvancedSunSky=off  SolarTime=11  TimeZone=-5  Day=21  Month=9  Year=2022  UseDaylightSavingTime=on  DSTStartDay=10  DSTStartMonth=3  DSTEndDay=3  DSTEndMonth=11  DSTSwitchHour=2  sensorTag=MainCamera1  sensorId=1  sensorName=MainCamera1  mountLoc=Origin  offsetFlag=off  tmountOffset=[0, 0, 0]  rmountOffset=[0, 0, 0]  HorizontalResolution=1280  VerticalResolution=720  HorizontalFOV=60  mountPoint=[0 0 0]  mountOrientation=[0 0 0]  aMode=0  ID=1  GeoTrigger=Inactive  ViewNameList={'Custom'}  ViewTranslationList={'[-6 0 2]'}  ViewRotationList={'[0 -15 0]'}
      settings: LibrarySourceBlock=aerolibsim3d/Simulation 3D Scene Configuration
  Subsystem : Subsystem
  speedM : Constant  Value=AngVel
  speedT : Constant  Value=AngVeltr
  wires:
  Demux/2 -> Simulation 3D Light Helicopter Pack/2
  states/1 -> Demux/1
  speedT/1 -> Subsystem/2(SpeedT)
  speedM/1 -> Subsystem/1(SpeedM)
  Simulation 3D Light Helicopter Pack/1 -> Simulation 3D Rotorcraft/1
  Add/1 -> Simulation 3D Light Helicopter Pack/1
  Subsystem/2(Position Blade 2) -> Simulation 3D Light Helicopter Pack/4
  Constant10/1 -> Add/1
  Simulation 3D Light Helicopter Pack/2 -> Simulation 3D Rotorcraft/2
  Subsystem/1(Position Blade1) -> Simulation 3D Light Helicopter Pack/3
  Demux/1 -> Add/2

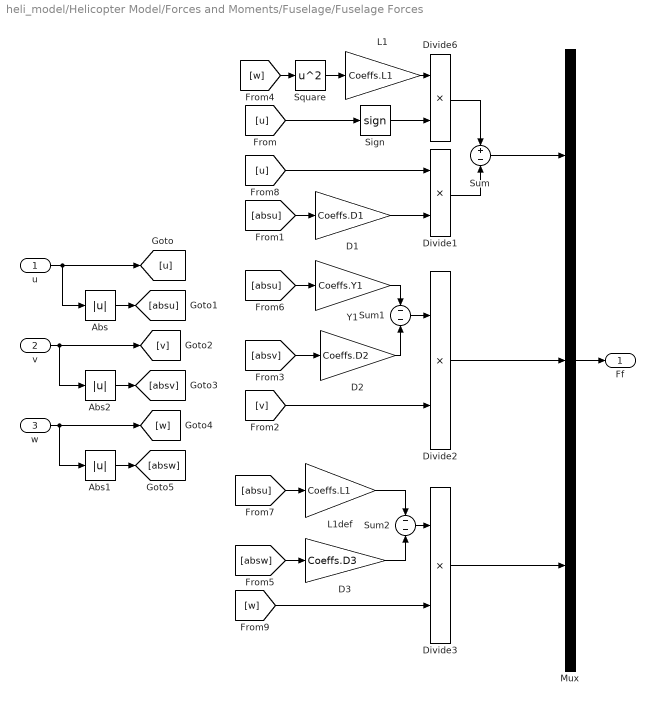
== system heli_model/Helicopter Model/Forces and Moments/Fuselage/Fuselage Forces ==
  u : Inport
  v : Inport  Port=2
  w : Inport  Port=3
  Abs : Abs  SaturateOnIntegerOverflow=off
  Abs1 : Abs  SaturateOnIntegerOverflow=off
  Abs2 : Abs  SaturateOnIntegerOverflow=off
  D1 : Gain  Gain=Coeffs.D1
  D2 : Gain  Gain=Coeffs.D2
  D3 : Gain  Gain=Coeffs.D3
  Divide{1..3,6} (4 alike) : Product  Inputs=**
  L1 : Gain  Gain=Coeffs.L1
  L1def : Gain  Gain=Coeffs.L1
  Mux : Mux  Inputs=3
  Sign : Signum
  Square : Math  Operator=square
  Sum : Sum  Inputs=+|-
  Sum1 : Sum  Inputs=-|-
  Sum2 : Sum  Inputs=-|-
  Y1 : Gain  Gain=Coeffs.Y1
  Ff : Outport
  wires:
  Sign/1 -> Divide6/2
  D2/1 -> Sum1/2
  Sum1/1 -> Divide2/1
  Divide6/1 -> Sum/1
  Divide2/1 -> Mux/2
  D3/1 -> Sum2/2
  L1def/1 -> Sum2/1
  Divide1/1 -> Sum/2
  Y1/1 -> Sum1/1
  Square/1 -> L1/1
  L1/1 -> Divide6/1
  Sum/1 -> Mux/1
  Divide3/1 -> Mux/3
  Sum2/1 -> Divide3/1
  Mux/1 -> Ff/1
  D1/1 -> Divide1/2
  [absu] -> D1/1
  [absu] -> Y1/1
  [absu] -> L1def/1
  [u] -> Sign/1
  [u] -> Divide1/1
  u/1 -> [u], Abs/1
  Abs/1 -> [absu]
  [w] -> Square/1
  [w] -> Divide3/2
  [absw] -> D3/1
  w/1 -> [w], Abs1/1
  Abs1/1 -> [absw]
  [v] -> Divide2/2
  [absv] -> D2/1
  v/1 -> [v], Abs2/1
  Abs2/1 -> [absv]

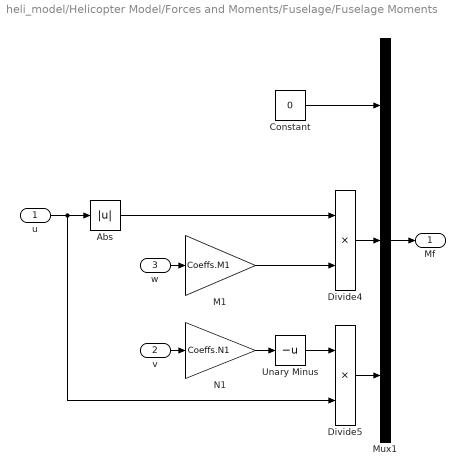
== system heli_model/Helicopter Model/Forces and Moments/Fuselage/Fuselage Moments ==
  u : Inport
  v : Inport  Port=2
  w : Inport  Port=3
  Abs : Abs  SaturateOnIntegerOverflow=off
  Constant : Constant  Value=0
  Divide4 : Product  Inputs=**
  Divide5 : Product  Inputs=**
  M1 : Gain  Gain=Coeffs.M1
  Mux1 : Mux  Inputs=3
  N1 : Gain  Gain=Coeffs.N1
  Unary Minus : UnaryMinus
  Mf : Outport
  wires:
  u/1 -> Divide5/2, Abs/1
  M1/1 -> Divide4/2
  N1/1 -> Unary Minus/1
  Mux1/1 -> Mf/1
  Divide5/1 -> Mux1/3
  Constant/1 -> Mux1/1
  v/1 -> N1/1
  Unary Minus/1 -> Divide5/1
  Divide4/1 -> Mux1/2
  w/1 -> M1/1
  Abs/1 -> Divide4/1

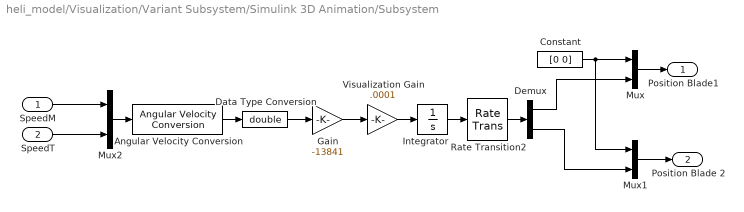
== system heli_model/Visualization/Variant Subsystem/Simulink 3D Animation/Subsystem ==
  SpeedM : Inport
  SpeedT : Inport  Port=2
  Angular Velocity Conversion : aerolibconvert2/Angular Velocity Conversion  IU=rad/s  OU=rpm
  Constant : Constant  Value=[0 0]  VectorParams1D=off
  Data Type Conversion : DataTypeConversion  OutDataTypeStr=double  SaturateOnIntegerOverflow=off  RndMeth=Floor
  Demux : Demux  Outputs=2
  Gain : Gain  Gain=-13841
  Integrator : Integrator  InitialCondition="[.1  .1]"  WrapState=on  WrappedStateUpperValue=2*pi  WrappedStateLowerValue=-2*pi
  Mux : Mux  Inputs=2
  Mux1 : Mux  Inputs=2
  Mux2 : Mux  Inputs=2
  Rate Transition2 : RateTransition
  Visualization Gain : Gain  Gain=.0001
  Position Blade1 : Outport  VectorParamsAs1DForOutWhenUnconnected=off
  Position Blade 2 : Outport  Port=2  VectorParamsAs1DForOutWhenUnconnected=off
  wires:
  Demux/2 -> Mux1/2
  Visualization Gain/1 -> Integrator/1
  Constant/1 -> Mux1/1, Mux/1
  Mux1/1 -> Position Blade 2/1
  Data Type Conversion/1 -> Gain/1
  Integrator/1 -> Rate Transition2/1
  Mux/1 -> Position Blade1/1
  Gain/1 -> Visualization Gain/1
  Demux/1 -> Mux/2
  Mux2/1 -> Angular Velocity Conversion/1
  Rate Transition2/1 -> Demux/1
  SpeedM/1 -> Mux2/1
  SpeedT/1 -> Mux2/2
  Angular Velocity Conversion/1 -> Data Type Conversion/1

== matlab function heli_model/LQR/MATLAB Function ==
  data: u input; K_table input; Vrefs input; K output
function K = getInterpolatedLQRcoeff(u,K_table,Vrefs)

    [r, c, ~] = size(K_table);
    K = zeros(r, c);

    for i = 1:r

        for j = 1:c
          
            value_vec = squeeze(K_table(i,j,:))'; 

            K(i,j) = interp1(Vrefs, value_vec, u, 'linear', 'extrap');
        end
        
    end

== matlab function heli_model/Autopilot/MATLAB Function ==
  data: x input; y input; Vx input; phi_ref output; Vy input; wp input; wp_index input; chi_d output; e_ct output; wp_index output
function [phi_ref, chi_d, e_ct, wp_index] = vf_guidance(x, y, Vx, Vy, wp, wp_index)

phi_ref = 0;
chi_d = atan2(Vy,Vx);
e_ct = 0;

k = 0.01;
k_phi = 0.6;
phi_max = deg2rad(35);

N = size(wp,1);

if wp_index >= N

    phi_ref = 0;
    chi_d = atan2(Vy,Vx);

    return
end

wp_current = wp(wp_index,:);
wp_next    = wp(wp_index+1,:);

dx = wp_next(1) - wp_current(1);
dy = wp_next(2) - wp_current(2);

L = sqrt(dx^2 + dy^2);

if L < 1e-6
    return
end

tx = dx / L;
ty = dy / L;

proj = (x - wp_current(1))*tx + (y - wp_current(2))*ty;

proj = max(0, min(proj, L));

if proj > L - 100 && wp_index < N-1

    wp_index = wp_index + 1;

    return
end

chi_path = atan2(ty, tx);

p_proj = wp_current + proj*[tx ty];

e_ct = -sin(chi_path)*(x - p_proj(1)) + cos(chi_path)*(y - p_proj(2));

chi_d = chi_path - atan2(k * e_ct,1);

chi_d = wrapToPi(chi_d);

chi = atan2(Vy, Vx);

e_chi = wrapToPi(chi_d - chi);

phi_ref = k_phi * e_chi;

phi_ref = max(min(phi_ref, phi_max), -phi_max);

end

== matlab function heli_model/Environment/stop ==
  data: u input; y output
function y = STOP(u)

y = false;

if u == 1
    disp('ÇAKILDI.');
    y = true;
end
